simulink model "xddd"  (R2023b)
settings: Solver=VariableStepAuto  StartTime=0.0  StopTime=10.0  RelTol=1e-3
settings Model: Creator=Admin  LastModifiedBy=Admin

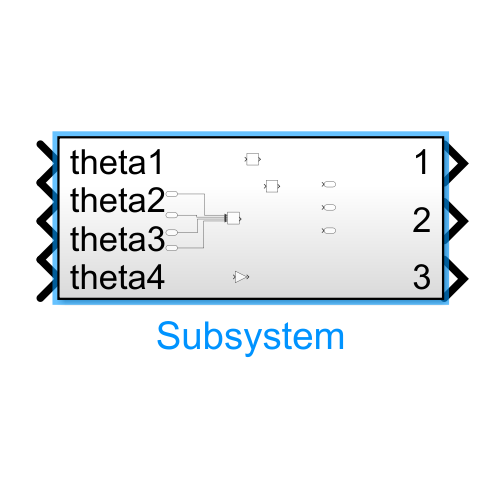
[thumbnail: Simulink's stored preview of the top-level diagram]
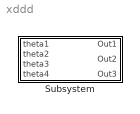
== system xddd ==
  Subsystem : Subsystem

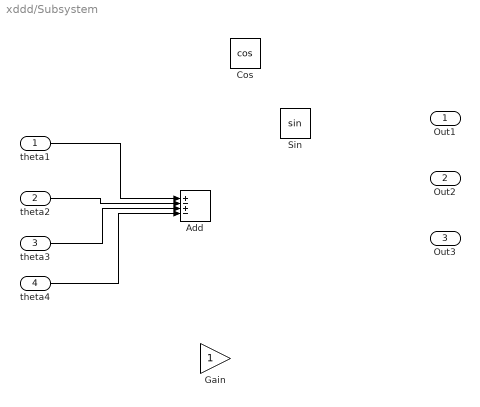
== system xddd/Subsystem ==
  theta1 : Inport
  theta2 : Inport  Port=2
  theta3 : Inport  Port=3
  theta4 : Inport  Port=4
  Add : Sum  Inputs=+-+-
  Cos : Trigonometry  Operator=cos
  Gain : Gain
  Sin : Trigonometry
  Out1 : Outport
  Out2 : Outport  Port=2
  Out3 : Outport  Port=3
  wires:
  theta1/1 -> Add/1
  theta2/1 -> Add/2
  theta3/1 -> Add/3
  theta4/1 -> Add/4
